simulink model "R_RC_EqCircuitMdl"  (R2019b)
settings: Solver=FixedStepAuto  StartTime=0.0  StopTime=tfinal  FixedStep=deltaT  RelTol=1e-3
InitFcn:
  | Init_Eq_Circuit_Model;
StopFcn:
  | ECM_Data_Processing;
values from neighbouring files (symbols this model uses):
  C1 = tau./R1    [Init_Eq_Circuit_Model.m]
  model =     [OCV0.mat]    (also in OCVrel.mat; SOC.mat)
  Q = mean(model.QParam)    [Init_Eq_Circuit_Model.m]
  R0 = (model.R0Param)    [Init_Eq_Circuit_Model.m]
  R1 = (model.RParam)    [Init_Eq_Circuit_Model.m]
  T = 25    [Init_Eq_Circuit_Model.m]
  temperatures = model.temps    [Init_Eq_Circuit_Model.m]
  Vc0 = 0    [Init_Eq_Circuit_Model.m]
  z0 = 1    [Init_Eq_Circuit_Model.m]
settings Model: Creator=miloshstojcic  LastModifiedBy=miloshstojcic

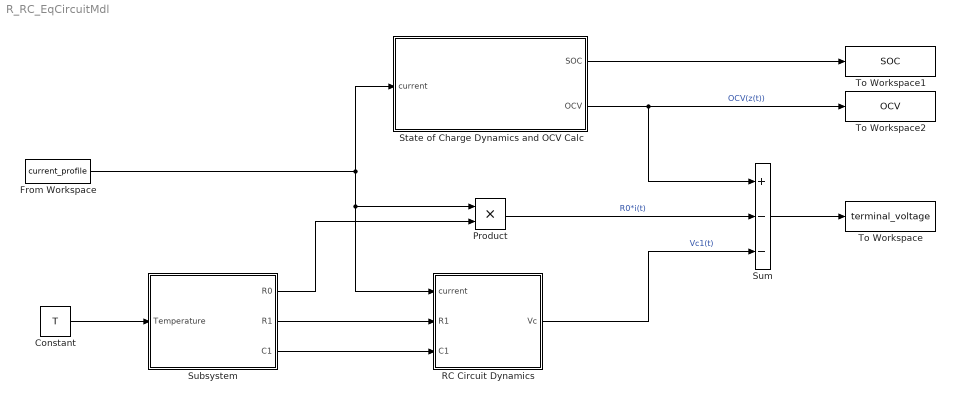
== system R_RC_EqCircuitMdl ==
  Constant : Constant  Value=T
  From Workspace : FromWorkspace  VariableName=current_profile  SampleTime=0
  Product : Product
  RC Circuit Dynamics : Subsystem
  State of Charge Dynamics and OCV Calc : Subsystem
  Subsystem : Subsystem
  Sum : Sum  Inputs=+--
  To Workspace : ToWorkspace  VariableName=terminal_voltage  SampleTime=-1
      settings: Save2DSignal=2-D array (concatenate along first dimension)
  To Workspace1 : ToWorkspace  VariableName=SOC  SampleTime=-1
      settings: Save2DSignal=2-D array (concatenate along first dimension)
  To Workspace2 : ToWorkspace  VariableName=OCV  SampleTime=-1
      settings: Save2DSignal=2-D array (concatenate along first dimension)
  wires:
  Constant/1 -> Subsystem/1(Temperature)
  Subsystem/2(R1) -> RC Circuit Dynamics/2(R1)
  Subsystem/3(C1) -> RC Circuit Dynamics/3(C1)
  From Workspace/1 -> State of Charge Dynamics and OCV Calc/1(current), Product/1, RC Circuit Dynamics/1(current)
  Subsystem/1(R0) -> Product/2
  State of Charge Dynamics and OCV Calc/2(OCV) -> Sum/1, To Workspace2/1  "OCV(z(t))"
  Product/1 -> Sum/2  "R0*i(t)"
  RC Circuit Dynamics/1(Vc) -> Sum/3  "Vc1(t)"
  Sum/1 -> To Workspace/1
  State of Charge Dynamics and OCV Calc/1(SOC) -> To Workspace1/1

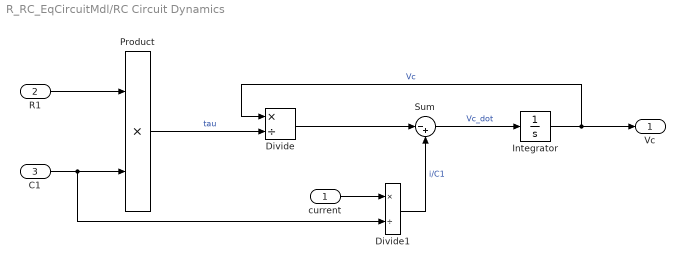
== system R_RC_EqCircuitMdl/RC Circuit Dynamics ==
  current : Inport
  R1 : Inport  Port=2
  C1 : Inport  Port=3
  Divide : Product  Inputs=*/
  Divide1 : Product  Inputs=*/
  Integrator : Integrator  InitialCondition=Vc0
  Product : Product
  Sum : Sum  Inputs=|-+
  Vc : Outport
  wires:
  C1/1 -> Divide1/2, Product/2
  R1/1 -> Product/1
  current/1 -> Divide1/1
  Divide1/1 -> Sum/2  "i/C1"
  Sum/1 -> Integrator/1  "Vc_dot"
  Integrator/1 -> Divide/1, Vc/1  "Vc"
  Product/1 -> Divide/2  "tau"
  Divide/1 -> Sum/1

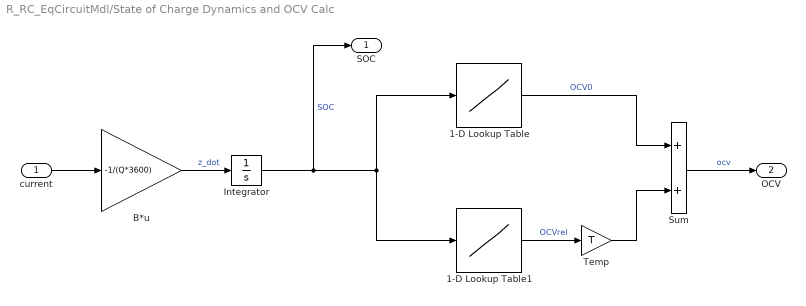
== system R_RC_EqCircuitMdl/State of Charge Dynamics and OCV Calc ==
  current : Inport
  1-D Lookup Table : Lookup_n-D  NumberOfTableDimensions=1  BreakpointsForDimension1=0:0.005:1  BreakpointsForDimension1FirstPoint=0  Table=model.OCV0  InternalRulePriority=Speed  RndMeth=Simplest  InputSameDT=on
  1-D Lookup Table1 : Lookup_n-D  NumberOfTableDimensions=1  BreakpointsForDimension1=[0:0.005:1]  BreakpointsForDimension1FirstPoint=0  Table=model.OCVrel  InternalRulePriority=Speed  RndMeth=Simplest  InputSameDT=on
  B*u : Gain  Gain=-1/(Q*3600)
  Integrator : Integrator  InitialCondition=z0
  Sum : Sum
  Temp : Gain  Gain=T
  SOC : Outport
  OCV : Outport  Port=2
  wires:
  current/1 -> B*u/1
  Sum/1 -> OCV/1  "ocv"
  B*u/1 -> Integrator/1  "z_dot"
  1-D Lookup Table1/1 -> Temp/1  "OCVrel"
  Temp/1 -> Sum/2
  1-D Lookup Table/1 -> Sum/1  "OCV0"
  Integrator/1 -> SOC/1, 1-D Lookup Table1/1, 1-D Lookup Table/1  "SOC"

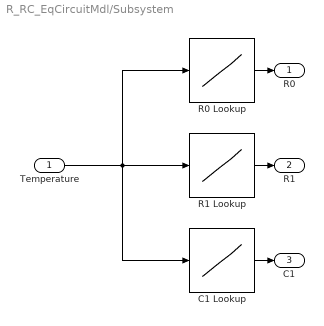
== system R_RC_EqCircuitMdl/Subsystem ==
  Temperature : Inport
  C1 Lookup : Lookup_n-D  NumberOfTableDimensions=1  BreakpointsForDimension1=temperatures  BreakpointsForDimension1FirstPoint=temperatures(1)  Table=C1  InternalRulePriority=Speed  RndMeth=Simplest  InputSameDT=on
  R0 Lookup : Lookup_n-D  NumberOfTableDimensions=1  BreakpointsForDimension1=temperatures  BreakpointsForDimension1FirstPoint=temperatures(1)  Table=R0  InternalRulePriority=Speed  RndMeth=Simplest  InputSameDT=on
  R1 Lookup : Lookup_n-D  NumberOfTableDimensions=1  BreakpointsForDimension1=temperatures  BreakpointsForDimension1FirstPoint=temperatures(1)  Table=R1  InternalRulePriority=Speed  RndMeth=Simplest  InputSameDT=on
  R0 : Outport
  R1 : Outport  Port=2
  C1 : Outport  Port=3
  wires:
  R0 Lookup/1 -> R0/1
  R1 Lookup/1 -> R1/1
  C1 Lookup/1 -> C1/1
  Temperature/1 -> R0 Lookup/1, R1 Lookup/1, C1 Lookup/1
